simulink model "chapter2_example_jd"  (R2016b)
settings: Solver=VariableStepAuto  StartTime=0.0  StopTime=10.0  RelTol=1e-3
PreLoadFcn:
  | load PI_output;
settings Model: Creator=training-ah  LastModifiedBy=training-ah
settings DataIOCC: ExternalInput=[PI_output_time, PI_output_data]  LoadExternalInput=on  SaveFormat=Array

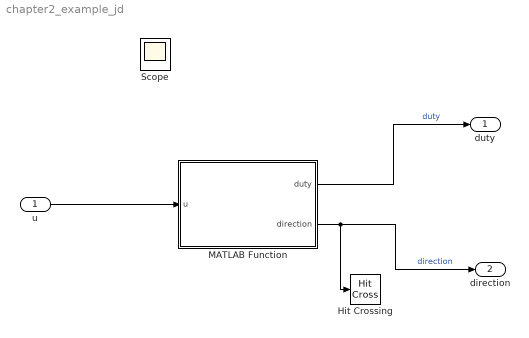
== system chapter2_example_jd ==
  u : Inport
  Hit Crossing : HitCross  ShowOutputPort=off
  MATLAB Function : MATLAB Function  TreatAsAtomicUnit=on
  duty : Outport
  direction : Outport  Port=2
  Scope : Scope
  wires:
  u/1 -> MATLAB Function/1(u)
  MATLAB Function/1(duty) -> duty/1  "duty"
  MATLAB Function/2(direction) -> direction/1, Hit Crossing/1  "direction"

== matlab function chapter2_example_jd/MATLAB Function ==
  data: u input; duty output; direction output
function [duty, direction] = u2dd(u)
% Set the direction and duty = abs(u)

if (u>=0)
    duty = u;
    direction = 1;
else
    duty = -u;
    direction = -1;
end

% Saturate duty cycle to 1
if duty > 1
    duty = 1;
end

y = u;
